simulink model "segmentCalcNeg"  (R2019a)
settings: Solver=VariableStepAuto  StartTime=0  StopTime=inf  FixedStep=1e-3  MaxStep=1e-3  RelTol=1e-3
values from neighbouring files (symbols this model uses):
  apexVelocity = flippedVel(n)    [Untitled.m]    (also in calcSegments.m = apexData.velocity(n,2); testInit.m)
  currentDistance = (flippedLocs(n) - 1) * init.ptDistance    [Untitled.m]    (also in calcSegments.m = (apexData.locs(n,1) - 1) * init.ptDistance; testInit.m)
  flippedCourse = flip(course)    [Untitled.m]    (also in calcSegments.m; testInit.m)
  init =     [course_data_0_1m.mat]
  stoppingDistance = (flippedLocs(n+1) - 1) * init.ptDistance    [Untitled.m]    (also in calcSegments.m = (apexData.locs(n+1,1) - 1) * init.ptDistance; testInit.m)
  TrackLength = 1161.1    [course_data_0_1m.mat]    (also in course_data_0_5m.mat = 1161; course_data_1m.mat = 1161; sortingPoints.m = (length(courseSorted)-1) * evalin('base', 'init.ptDistance'))
libraries: simulink x1
settings Model: Creator=Frieder Uerlings  LastModifiedBy=Frieder Uerlings
settings SolverCC: ZeroCrossControl=DisableAll  AlgebraicLoopSolver=LineSearch

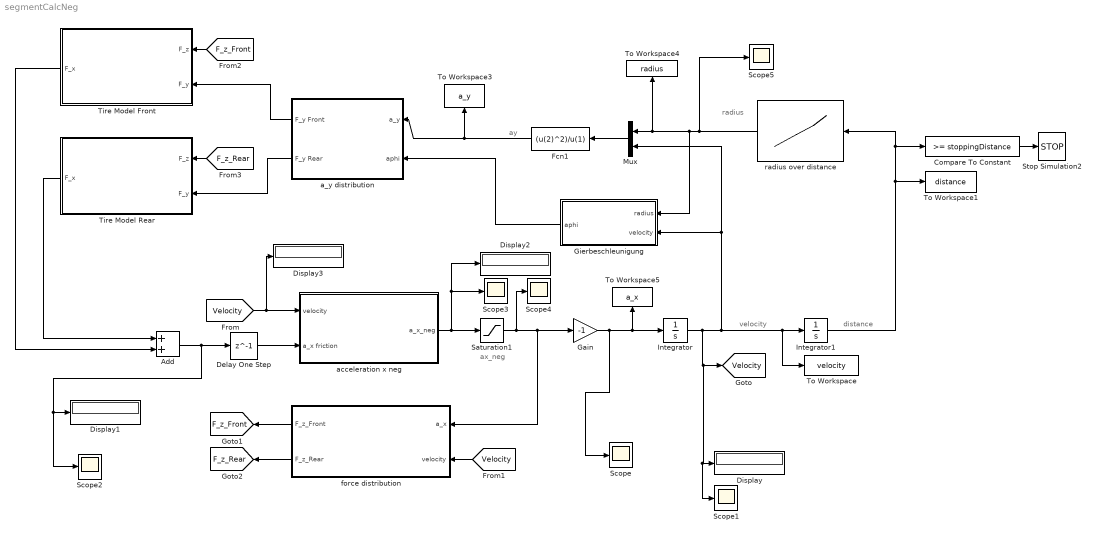
== system segmentCalcNeg ==
  note: velocity
  note: distance
  note: ay
  note: radius
  note: ax_neg
  Add : Sum
  Compare To Constant : simulink/Logic and Bit Operations/Compare To Constant  relop=>=  const=stoppingDistance  OutDataTypeStr=boolean
  Delay One Step : Delay  DelayLength=1
  Display{,1..3} (4 alike) : Display
  Fcn1 : Fcn  Expr=(u(2)^2)/u(1)
  Gain : Gain  Gain=-1
  Gierbeschleunigung : Subsystem
  Integrator : Integrator  InitialCondition=apexVelocity
  Integrator1 : Integrator  InitialCondition=currentDistance
  Mux : Mux  Inputs=2
  Saturation1 : Saturate  UpperLimit=0  LowerLimit=-inf  ZeroCross=off
  Scope{,1..5} (6 alike) : Scope
  Stop Simulation2 : Stop
  Tire Model Front : Subsystem
  Tire Model Rear : Subsystem
  To Workspace : ToWorkspace  VariableName=velocity  SampleTime=-1
  To Workspace1 : ToWorkspace  VariableName=distance  SampleTime=-1
  To Workspace3 : ToWorkspace  VariableName=a_y  SampleTime=-1
  To Workspace4 : ToWorkspace  VariableName=radius  SampleTime=-1
  To Workspace5 : ToWorkspace  VariableName=a_x  SampleTime=-1
  a_y distribution : Subsystem
  acceleration x neg : Subsystem
  force distribution : Subsystem
  radius over distance : Lookup_n-D  NumberOfTableDimensions=1  BreakpointsForDimension1=[0:init.ptDistance:TrackLength]  Table=flippedCourse(:,3)  InternalRulePriority=Speed  RndMeth=Simplest  InputSameDT=on
  tag scope: F_z_Front=global, F_z_Rear=global, Velocity=global
  wires:
  radius over distance/1 -> Scope5/1, Gierbeschleunigung/1(radius), Mux/1, To Workspace4/1
  Compare To Constant/1 -> Stop Simulation2/1
  Tire Model Rear/1(F_x) -> Add/1
  [F_z_Front] -> Tire Model Front/1(F_z)
  acceleration x neg/1("a_x_neg ") -> Scope3/1, Display2/1, Saturation1/1
  Gierbeschleunigung/1(aphi) -> a_y distribution/2("aphi ")
  force distribution/2("F_z_Rear ") -> [F_z_Rear]
  a_y distribution/1("F_y Front ") -> Tire Model Front/2(F_y)
  [Velocity] -> Display3/1, acceleration x neg/1(velocity)
  force distribution/1(F_z_Front) -> [F_z_Front]
  a_y distribution/2("F_y Rear ") -> Tire Model Rear/2(F_y)
  Fcn1/1 -> a_y distribution/1("a_y "), To Workspace3/1
  Integrator1/1 -> To Workspace1/1, Compare To Constant/1, radius over distance/1
  [Velocity] -> force distribution/2("velocity ")
  Mux/1 -> Fcn1/1
  [F_z_Rear] -> Tire Model Rear/1(F_z)
  Tire Model Front/1(F_x) -> Add/2
  Saturation1/1 -> Scope4/1, Gain/1, force distribution/1("a_x ")
  Gain/1 -> Scope/1, To Workspace5/1, Integrator/1
  Add/1 -> Delay One Step/1, Scope2/1, Display1/1
  Integrator/1 -> Scope1/1, Display/1, [Velocity], Gierbeschleunigung/2("velocity "), Mux/2, To Workspace/1, Integrator1/1
  Delay One Step/1 -> acceleration x neg/2(a_x friction)

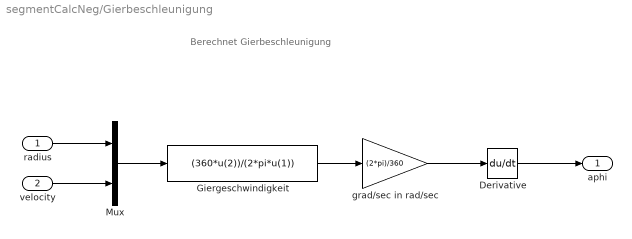
== system segmentCalcNeg/Gierbeschleunigung ==
  note: Berechnet Gierbeschleunigung
  radius : Inport
  "velocity " : Inport  Port=2
  Derivative : Derivative
  Giergeschwindigkeit : Fcn  Expr=(360*u(2))/(2*pi*u(1))
  Mux : Mux  Inputs=2
  grad/sec in rad/sec : Gain  Gain=(2*pi)/360
  aphi : Outport
  wires:
  radius/1 -> Mux/1
  "velocity "/1 -> Mux/2
  Mux/1 -> Giergeschwindigkeit/1
  Giergeschwindigkeit/1 -> grad/sec in rad/sec/1
  grad/sec in rad/sec/1 -> Derivative/1
  Derivative/1 -> aphi/1

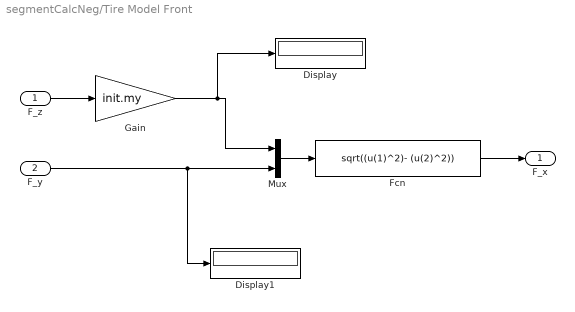
== system segmentCalcNeg/Tire Model Front ==
  F_z : Inport
  F_y : Inport  Port=2
  Display : Display
  Display1 : Display
  Fcn : Fcn  Expr=sqrt((u(1)^2)- (u(2)^2))
  Gain : Gain  Gain=init.my
  Mux : Mux  Inputs=2
  F_x : Outport
  wires:
  F_z/1 -> Gain/1
  Fcn/1 -> F_x/1
  Mux/1 -> Fcn/1
  Gain/1 -> Display/1, Mux/1
  F_y/1 -> Display1/1, Mux/2

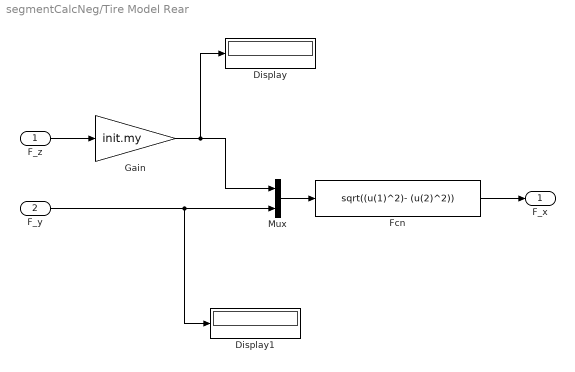
== system segmentCalcNeg/Tire Model Rear ==
  F_z : Inport
  F_y : Inport  Port=2
  Display : Display
  Display1 : Display
  Fcn : Fcn  Expr=sqrt((u(1)^2)- (u(2)^2))
  Gain : Gain  Gain=init.my
  Mux : Mux  Inputs=2
  F_x : Outport
  wires:
  F_y/1 -> Display1/1, Mux/2
  Gain/1 -> Display/1, Mux/1
  Mux/1 -> Fcn/1
  Fcn/1 -> F_x/1
  F_z/1 -> Gain/1

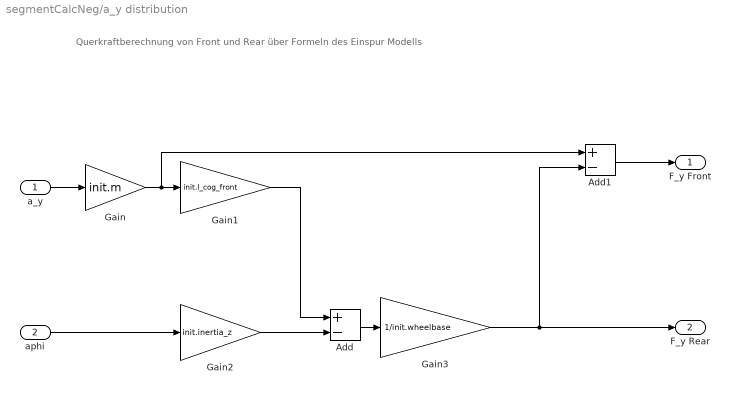
== system segmentCalcNeg/a_y distribution ==
  note: Querkraftberechnung von Front und Rear über Formeln des Einspur Modells
  "a_y " : Inport
  "aphi " : Inport  Port=2
  Add : Sum  Inputs=+-
  Add1 : Sum  Inputs=+-
  Gain : Gain  Gain=init.m
  Gain1 : Gain  Gain=init.l_cog_front
  Gain2 : Gain  Gain=init.inertia_z
  Gain3 : Gain  Gain=1/init.wheelbase
  "F_y Front " : Outport
  "F_y Rear " : Outport  Port=2
  wires:
  "a_y "/1 -> Gain/1
  Gain/1 -> Add1/1, Gain1/1
  Gain1/1 -> Add/1
  Gain2/1 -> Add/2
  "aphi "/1 -> Gain2/1
  Add/1 -> Gain3/1
  Add1/1 -> "F_y Front "/1
  Gain3/1 -> Add1/2, "F_y Rear "/1

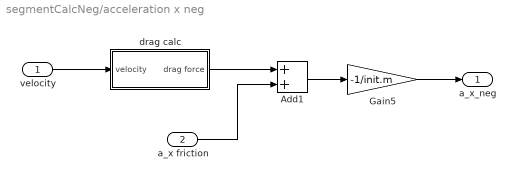
== system segmentCalcNeg/acceleration x neg ==
  velocity : Inport
  a_x friction : Inport  Port=2
  Add1 : Sum
  Gain5 : Gain  Gain=-1/init.m
  drag calc : Subsystem
  "a_x_neg " : Outport
  wires:
  drag calc/1("drag force ") -> Add1/1
  a_x friction/1 -> Add1/2
  velocity/1 -> drag calc/1(velocity)
  Gain5/1 -> "a_x_neg "/1
  Add1/1 -> Gain5/1

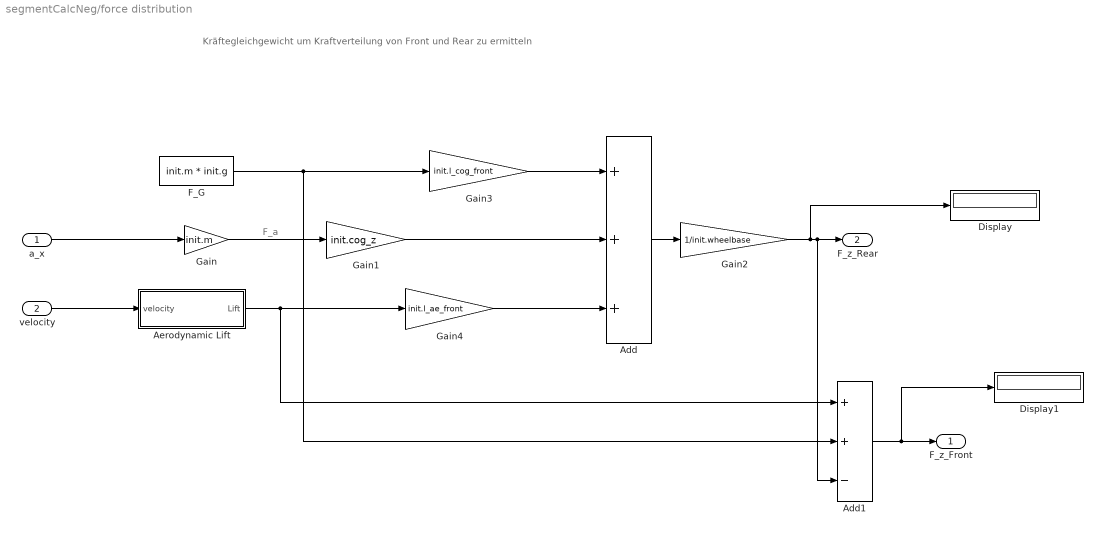
== system segmentCalcNeg/force distribution ==
  note: Kräftegleichgewicht um Kraftverteilung von Front und Rear zu ermitteln
  note: F_a
  "a_x " : Inport
  "velocity " : Inport  Port=2
  Add : Sum  Inputs=+++
  Add1 : Sum  Inputs=++-
  Aerodynamic Lift : Subsystem
  Display : Display
  Display1 : Display
  "F_G " : Constant  Value=init.m * init.g
  Gain : Gain  Gain=init.m
  Gain1 : Gain  Gain=init.cog_z
  Gain2 : Gain  Gain=1/init.wheelbase
  Gain3 : Gain  Gain=init.l_cog_front
  Gain4 : Gain  Gain=init.l_ae_front
  F_z_Front : Outport
  "F_z_Rear " : Outport  Port=2
  wires:
  "a_x "/1 -> Gain/1
  "F_G "/1 -> Add1/2, Gain3/1
  Gain3/1 -> Add/1
  Gain/1 -> Gain1/1
  "velocity "/1 -> Aerodynamic Lift/1(velocity)
  Aerodynamic Lift/1(Lift) -> Gain4/1, Add1/1
  Gain1/1 -> Add/2
  Gain4/1 -> Add/3
  Add/1 -> Gain2/1
  Gain2/1 -> Display/1, Add1/3, "F_z_Rear "/1
  Add1/1 -> Display1/1, F_z_Front/1

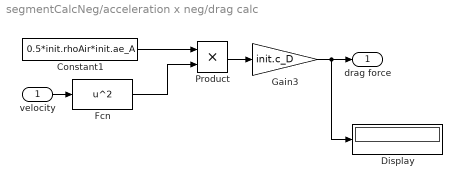
== system segmentCalcNeg/acceleration x neg/drag calc ==
  velocity : Inport
  Constant1 : Constant  Value=0.5*init.rhoAir*init.ae_A
  Display : Display
  Fcn : Fcn  Expr=u^2
  Gain3 : Gain  Gain=init.c_D
  Product : Product
  "drag force " : Outport
  wires:
  Constant1/1 -> Product/1
  velocity/1 -> Fcn/1
  Fcn/1 -> Product/2
  Product/1 -> Gain3/1
  Gain3/1 -> Display/1, "drag force "/1

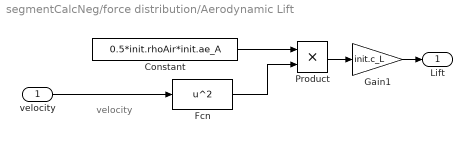
== system segmentCalcNeg/force distribution/Aerodynamic Lift ==
  note: velocity
  velocity : Inport
  Constant : Constant  Value=0.5*init.rhoAir*init.ae_A
  Fcn : Fcn  Expr=u^2
  Gain1 : Gain  Gain=init.c_L
  Product : Product
  Lift : Outport
  wires:
  Fcn/1 -> Product/2
  velocity/1 -> Fcn/1
  Constant/1 -> Product/1
  Product/1 -> Gain1/1
  Gain1/1 -> Lift/1
